simulink model "nonlin_3d"  (R2023a)
settings: Solver=ode1  StartTime=0  StopTime=400  FixedStep=0.002  RelTol=1e-3
values from neighbouring files (symbols this model uses):
  B1 = [-kQ, -kQ, kQ, kQ ... (first row only)    [simulate_hover.m]
  B2 = [0, 0, 0 ... (first row only)    [simulate_hover.m]
  beta3d = 0.9    [loadResultData.m]    (also in simulate_hover.m; temp.m)
  cycleGain = 0.2    [simulate_hover.m]    (also in temp.m = 1)
  epsilon3d = 1    [loadResultData.m]    (also in simulate_hover.m; temp.m)
  I_xx = 0.0522    [simulate_hover.m]
  I_yy = 0.0522    [simulate_hover.m]
  I_zz = 0.1104    [simulate_hover.m]
  K = lqi(sys, Q, R)    [simulate_hover.m]
  k3d = 1.65    [loadResultData.m]    (also in simulate_hover.m; temp.m)
  kfr_p = 0.4*u2line/x5line    (= 0.285774113641)    [simulate_hover.m]
  kfr_r = 0.4*u1line/x4line    (= 0.285774113641)    [simulate_hover.m]
  kfr_y = 0.4*u3line/x6line    (= 0.0880063173321)    [simulate_hover.m]
  sigma = 0    [simulate_hover.m]
  velMax = 100*60*pi/180    (= 104.71975512)    [simulate_hover.m]
  VMAX_AMP = 24    [setup_lab_hover.m]    (also in simulate_hover.m)
  wcf = 2 * pi * 20    (= 125.663706144)    [setup_lab_hover.m]    (also in simulate_hover.m)
  zetaf = 0.6    [setup_lab_hover.m]    (also in simulate_hover.m)
undefined symbols (not defined in the file or in its folder): DG
libraries: simulink_extras x1, dspsrcs4 x1
settings Model: Creator=kille  LastModifiedBy=Jacob

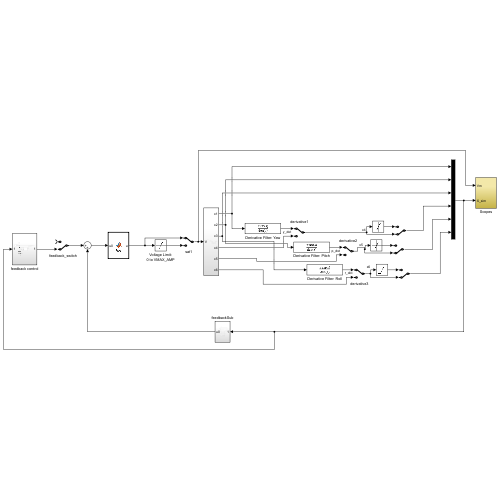
[thumbnail: Simulink's stored preview of the top-level diagram]
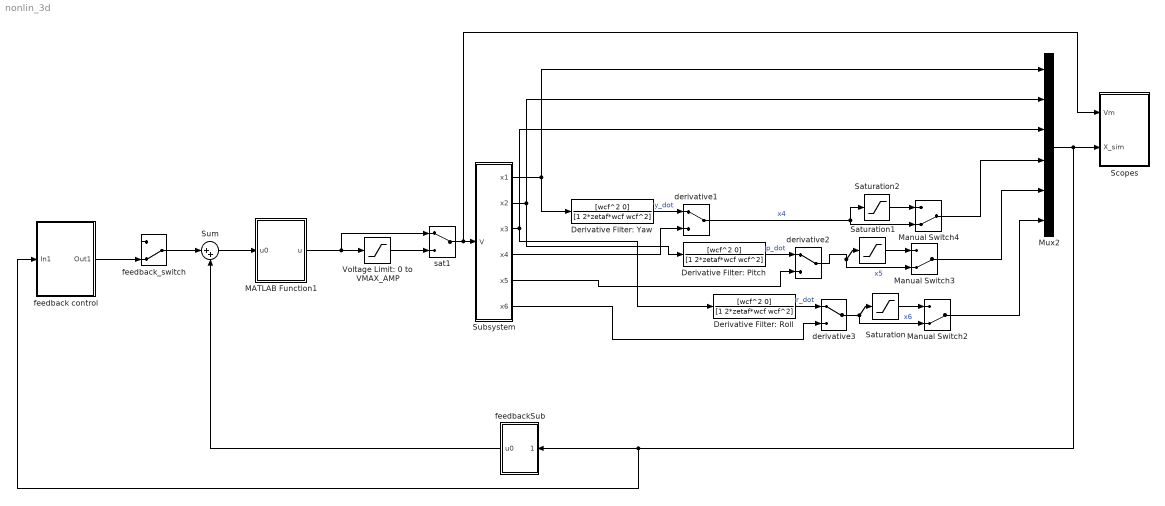
== system nonlin_3d ==
  Derivative Filter: Pitch : TransferFcn  Numerator=[wcf^2 0]  Denominator=[1 2*zetaf*wcf wcf^2]
  Derivative Filter: Roll : TransferFcn  Numerator=[wcf^2 0]  Denominator=[1 2*zetaf*wcf wcf^2]
  Derivative Filter: Yaw : TransferFcn  Numerator=[wcf^2 0]  Denominator=[1 2*zetaf*wcf wcf^2]
  MATLAB Function1 : MATLAB Function  TreatAsAtomicUnit=on
  Manual Switch2 : ManualSwitch  CurrentSetting=0
  Manual Switch3 : ManualSwitch  CurrentSetting=0
  Manual Switch4 : ManualSwitch  CurrentSetting=0
  Mux2 : Mux  Inputs=6
  Saturation : Saturate  UpperLimit=velMax  LowerLimit=-velMax
  Saturation1 : Saturate  UpperLimit=velMax  LowerLimit=-velMax
  Saturation2 : Saturate  UpperLimit=velMax  LowerLimit=-velMax
  Scopes : Subsystem
  Subsystem : Subsystem
  Sum : Sum  Inputs=|++
  Voltage Limit: 0 to VMAX_AMP : Saturate  UpperLimit=VMAX_AMP  LowerLimit=0
  derivative1 : ManualSwitch
  derivative2 : ManualSwitch
  derivative3 : ManualSwitch
  feedback control : Subsystem
  feedbackSub : Subsystem
  feedback_switch : ManualSwitch  CurrentSetting=0
  sat1 : ManualSwitch
  wires:
  Derivative Filter: Yaw/1 -> derivative1/1  "y_dot"
  Derivative Filter: Pitch/1 -> derivative2/1  "p_dot"
  Derivative Filter: Roll/1 -> derivative3/1  "r_dot"
  Subsystem/1(x1) -> Mux2/1, Derivative Filter: Yaw/1
  Subsystem/4(x4) -> derivative1/2
  Subsystem/2(x2) -> Derivative Filter: Pitch/1, Mux2/2
  Subsystem/5(x5) -> derivative2/2
  Subsystem/6(x6) -> derivative3/2
  Subsystem/3(x3) -> Mux2/3, Derivative Filter: Roll/1
  Manual Switch4/1 -> Mux2/4
  Manual Switch2/1 -> Mux2/6
  Manual Switch3/1 -> Mux2/5
  Saturation/1 -> Manual Switch2/1
  derivative3/1 -> Manual Switch2/2, Saturation/1  "x6"
  Saturation1/1 -> Manual Switch3/1
  derivative2/1 -> Manual Switch3/2, Saturation1/1  "x5"
  Saturation2/1 -> Manual Switch4/1
  derivative1/1 -> Saturation2/1, Manual Switch4/2  "x4"
  MATLAB Function1/1(u) -> sat1/1, Voltage Limit: 0 to VMAX_AMP/1
  sat1/1 -> Scopes/1(Vm), Subsystem/1(V)
  Voltage Limit: 0 to VMAX_AMP/1 -> sat1/2
  feedback control/1(Out1) -> feedback_switch/2
  Mux2/1 -> feedback control/1(In1), feedbackSub/1(Input), Scopes/2(X_sim)
  feedback_switch/1 -> Sum/1
  Sum/1 -> MATLAB Function1/1(u0)
  feedbackSub/1(u0) -> Sum/2

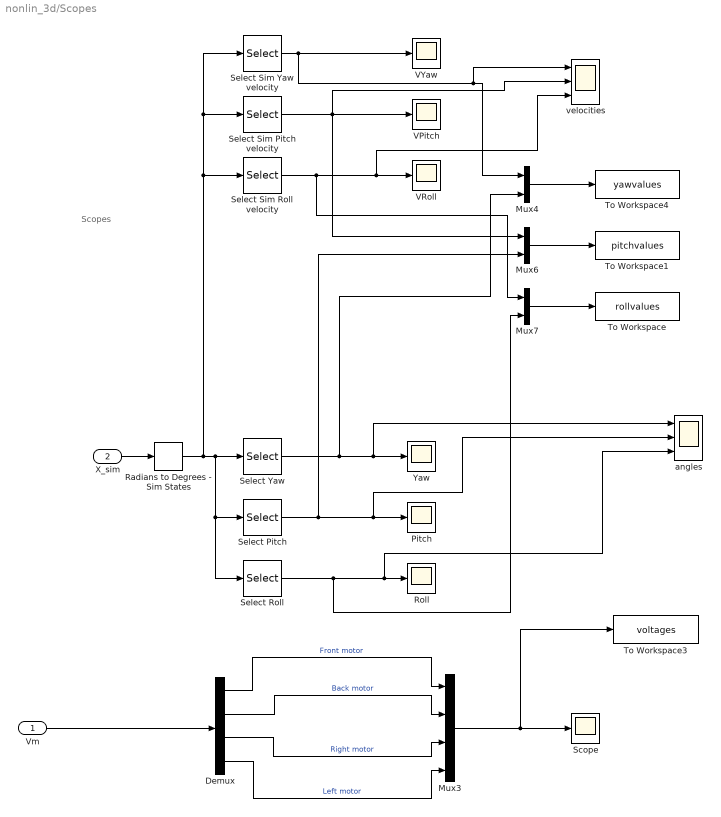
== system nonlin_3d/Scopes ==
  note: Scopes
  Vm : Inport
  X_sim : Inport  Port=2
  Demux : Demux
  Mux3 : Mux
  Mux4 : Mux  Inputs=2
  Mux6 : Mux  Inputs=2
  Mux7 : Mux  Inputs=2
  Pitch : Scope
  Radians to Degrees - Sim States : simulink_extras/Transformations/Radians to Degrees
  Roll : Scope
  Scope : Scope
  Select Pitch : Selector  InputPortWidth=6  IndexOptions=Index vector (dialog)  Indices=2  OutputSizes=1
  Select Roll : Selector  InputPortWidth=6  IndexOptions=Index vector (dialog)  Indices=3  OutputSizes=1
  Select Sim Pitch velocity : Selector  InputPortWidth=6  IndexOptions=Index vector (dialog)  Indices=5  OutputSizes=1
  Select Sim Roll velocity : Selector  InputPortWidth=6  IndexOptions=Index vector (dialog)  Indices=6  OutputSizes=1
  Select Sim Yaw velocity : Selector  InputPortWidth=6  IndexOptions=Index vector (dialog)  Indices=4  OutputSizes=1
  Select Yaw : Selector  InputPortWidth=6  IndexOptions=Index vector (dialog)  Indices=1  OutputSizes=1
  To Workspace : ToWorkspace  VariableName=rollvalues  SampleTime=-1
  To Workspace1 : ToWorkspace  VariableName=pitchvalues  SampleTime=-1
  To Workspace3 : ToWorkspace  VariableName=voltages  SampleTime=-1
  To Workspace4 : ToWorkspace  VariableName=yawvalues  SampleTime=-1
  VPitch : Scope
  VRoll : Scope
  VYaw : Scope
  Yaw : Scope
  angles : Scope  NumInputPorts=3
  velocities : Scope  NumInputPorts=3
  wires:
  Select Roll/1 -> angles/3, Roll/1, Mux7/2
  Radians to Degrees - Sim States/1 -> Select Sim Roll velocity/1, Select Sim Pitch velocity/1, Select Sim Yaw velocity/1, Select Roll/1, Select Pitch/1, Select Yaw/1
  Select Pitch/1 -> angles/2, Pitch/1, Mux6/2
  X_sim/1 -> Radians to Degrees - Sim States/1
  Demux/1 -> Mux3/1  "Front motor"
  Demux/2 -> Mux3/2  "Back motor"
  Demux/3 -> Mux3/3  "Right motor"
  Demux/4 -> Mux3/4  "Left motor"
  Vm/1 -> Demux/1
  Select Sim Yaw velocity/1 -> VYaw/1, velocities/1, Mux4/1
  Select Sim Roll velocity/1 -> velocities/3, VRoll/1, Mux7/1
  Select Sim Pitch velocity/1 -> Mux6/1, velocities/2, VPitch/1
  Mux4/1 -> To Workspace4/1
  Mux6/1 -> To Workspace1/1
  Mux7/1 -> To Workspace/1
  Mux3/1 -> To Workspace3/1, Scope/1
  Select Yaw/1 -> angles/1, Yaw/1, Mux4/2

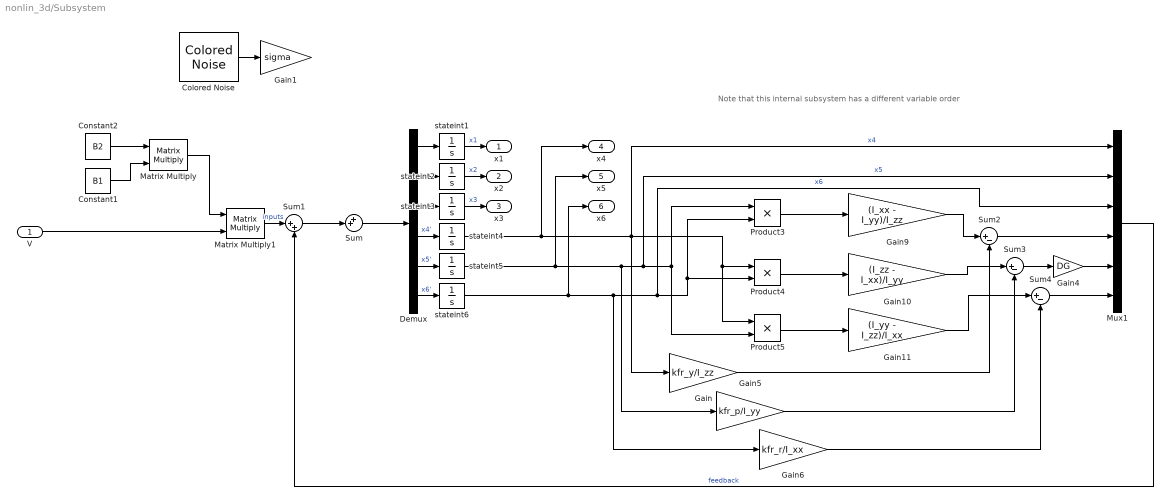
== system nonlin_3d/Subsystem ==
  note: Note that this internal subsystem has a different variable order
  V : Inport
  Colored Noise : dspsrcs4/Colored Noise  Color=white  InverseFrequencyPower=1  BoundedOutput=off  NumChannels=6  OutputDataType=double  SamplesPerFrame=1  SampleTime=1  RandomStream=mt19937ar with seed  Seed=67  SimulateUsing=Interpreted execution
  Constant1 : Constant  Value=B1
  Constant2 : Constant  Value=B2
  Demux : Demux  Outputs=6
  Gain : Gain  Gain=kfr_y/I_zz
  Gain1 : Gain  Gain=sigma
  Gain10 : Gain  Gain=(I_zz - I_xx)/I_yy
  Gain11 : Gain  Gain=(I_yy - I_zz)/I_xx
  Gain4 : Gain  Gain=DG
  Gain5 : Gain  Gain=kfr_p/I_yy
  Gain6 : Gain  Gain=kfr_r/I_xx
  Gain9 : Gain  Gain=(I_xx - I_yy)/I_zz
  Matrix Multiply : Product  Multiplication=Matrix(*)
  Matrix Multiply1 : Product  Multiplication=Matrix(*)
  Mux1 : Mux  Inputs=6
  Product3 : Product
  Product4 : Product
  Product5 : Product
  Sum : Sum  Inputs=++|
  Sum1 : Sum  Inputs=|++
  Sum2 : Sum  Inputs=|+-
  Sum3 : Sum  Inputs=|+-
  Sum4 : Sum  Inputs=|+-
  stateint{1,4..6} (4 alike) : Integrator
  stateint2 : Integrator  InitialCondition=0.00010472
  stateint3 : Integrator  InitialCondition=0.00010472
  x1 : Outport
  x2 : Outport  Port=2
  x3 : Outport  Port=3
  x4 : Outport  Port=4
  x5 : Outport  Port=5
  x6 : Outport  Port=6
  wires:
  Mux1/1 -> Sum1/2  "feedback"
  stateint5/1 -> x5/1, Gain5/1, Mux1/2, Product5/2, Product3/1  "x5"
  Matrix Multiply1/1 -> Sum1/1  "inputs"
  stateint4/1 -> x4/1, Gain/1, Mux1/1, Product5/1, Product4/1  "x4"
  Matrix Multiply/1 -> Matrix Multiply1/1
  V/1 -> Matrix Multiply1/2
  Sum2/1 -> Mux1/4
  Gain6/1 -> Sum4/2
  Demux/1 -> stateint1/1
  stateint6/1 -> x6/1, Gain6/1, Mux1/3, Product4/2, Product3/2  "x6"
  Demux/6 -> stateint6/1  "x6'"
  Product5/1 -> Gain11/1
  Demux/5 -> stateint5/1  "x5'"
  Demux/2 -> stateint2/1
  Gain11/1 -> Sum4/1
  Constant1/1 -> Matrix Multiply/2
  Demux/3 -> stateint3/1
  Gain9/1 -> Sum2/1
  Gain10/1 -> Sum3/1
  Constant2/1 -> Matrix Multiply/1
  Demux/4 -> stateint4/1  "x4'"
  Product4/1 -> Gain10/1
  stateint1/1 -> x1/1  "x1"
  stateint2/1 -> x2/1  "x2"
  stateint3/1 -> x3/1  "x3"
  Colored Noise/1 -> Gain1/1
  Sum1/1 -> Sum/2
  Sum/1 -> Demux/1
  Product3/1 -> Gain9/1
  Gain/1 -> Sum2/2
  Gain5/1 -> Sum3/2
  Sum3/1 -> Gain4/1
  Sum4/1 -> Mux1/6
  Gain4/1 -> Mux1/5

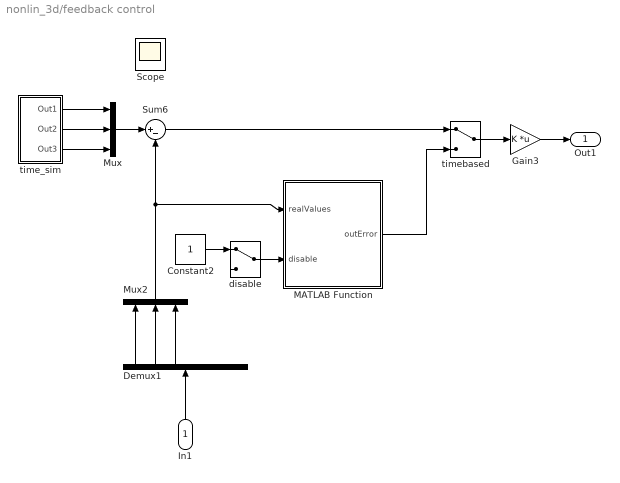
== system nonlin_3d/feedback control ==
  In1 : Inport
  Constant2 : Constant
  Demux1 : Demux  Outputs=6
  Gain3 : Gain  Gain=K  Multiplication=Matrix(K*u)
  MATLAB Function : MATLAB Function  TreatAsAtomicUnit=on
  Mux : Mux  Inputs=3
  Mux2 : Mux  Inputs=3
  Scope : Scope
  Sum6 : Sum  Inputs=|+-
  disable : ManualSwitch
  time_sim : Subsystem
  timebased : ManualSwitch
  Out1 : Outport
  wires:
  Demux1/2 -> Mux2/2
  Demux1/1 -> Mux2/1
  Demux1/3 -> Mux2/3
  In1/1 -> Demux1/1
  MATLAB Function/1(outError) -> timebased/2
  Sum6/1 -> timebased/1
  timebased/1 -> Gain3/1
  Gain3/1 -> Out1/1
  Mux2/1 -> MATLAB Function/1(realValues), Sum6/2
  disable/1 -> MATLAB Function/2(disable)
  Constant2/1 -> disable/1
  Mux/1 -> Sum6/1
  time_sim/1(Out1) -> Mux/1
  time_sim/2(Out2) -> Mux/2
  time_sim/3(Out3) -> Mux/3

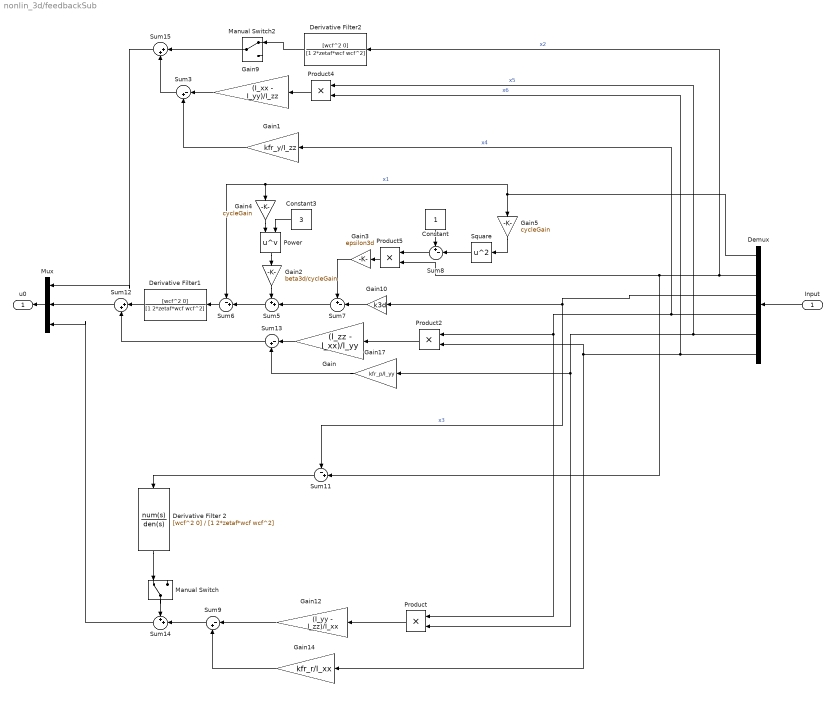
== system nonlin_3d/feedbackSub ==
  Input : Inport
  Constant : Constant
  Constant3 : Constant  Value=3
  Demux : Demux  Outputs=6
  Derivative Filter 2 : TransferFcn  Numerator=[wcf^2 0]  Denominator=[1 2*zetaf*wcf wcf^2]
  Derivative Filter1 : TransferFcn  Numerator=[wcf^2 0]  Denominator=[1 2*zetaf*wcf wcf^2]
  Derivative Filter2 : TransferFcn  Numerator=[wcf^2 0]  Denominator=[1 2*zetaf*wcf wcf^2]
  Gain : Gain  Gain=(I_zz - I_xx)/I_yy
  Gain1 : Gain  Gain=kfr_y/I_zz
  Gain10 : Gain  Gain=k3d
  Gain12 : Gain  Gain=(I_yy - I_zz)/I_xx
  Gain14 : Gain  Gain=kfr_r/I_xx
  Gain17 : Gain  Gain=kfr_p/I_yy
  Gain2 : Gain  Gain=beta3d/cycleGain
  Gain3 : Gain  Gain=epsilon3d
  Gain4 : Gain  Gain=cycleGain
  Gain5 : Gain  Gain=cycleGain
  Gain9 : Gain  Gain=(I_xx - I_yy)/I_zz
  Manual Switch : ManualSwitch
  Manual Switch2 : ManualSwitch
  Mux : Mux  Inputs=3
  Power : Math  Operator=pow
  Product{,2,4..5} (4 alike) : Product
  Square : Math  Operator=square
  Sum11 : Sum  Inputs=-+|
  Sum12 : Sum  Inputs=|++
  Sum13 : Sum  Inputs=|-+
  Sum14 : Sum  Inputs=++|
  Sum15 : Sum  Inputs=|++
  Sum3 : Sum  Inputs=|-+
  Sum5 : Sum  Inputs=++|
  Sum6 : Sum  Inputs=-+|
  Sum7 : Sum  Inputs=+-|
  Sum8 : Sum  Inputs=+-|
  Sum9 : Sum  Inputs=|-+
  u0 : Outport
  wires:
  Gain17/1 -> Sum13/2
  Sum13/1 -> Sum12/2
  Demux/4 -> Product/1, Product2/1, Gain1/1  "x4"
  Product2/1 -> Gain/1
  Demux/5 -> Product4/1, Product/2, Gain17/1  "x5"
  Product/1 -> Gain12/1
  Demux/6 -> Gain14/1, Product2/2, Product4/2  "x6"
  Manual Switch/1 -> Sum14/1
  Sum9/1 -> Sum14/2
  Gain12/1 -> Sum9/1
  Gain/1 -> Sum13/1
  Gain14/1 -> Sum9/2
  Sum12/1 -> Mux/2
  Derivative Filter 2/1 -> Manual Switch/1
  Sum14/1 -> Mux/3
  Input/1 -> Demux/1
  Demux/3 -> Gain10/1, Sum11/1  "x3"
  Product4/1 -> Gain9/1
  Gain9/1 -> Sum3/1
  Gain1/1 -> Sum3/2
  Gain3/1 -> Sum7/1
  Gain2/1 -> Sum5/1
  Constant/1 -> Sum8/1
  Constant3/1 -> Power/2
  Square/1 -> Sum8/2
  Sum8/1 -> Product5/1
  Gain10/1 -> Sum7/2
  Sum7/1 -> Sum5/2
  Sum5/1 -> Sum6/2
  Product5/1 -> Gain3/1
  Power/1 -> Gain2/1
  Manual Switch2/1 -> Sum15/1
  Demux/2 -> Derivative Filter2/1, Product5/2, Sum11/2  "x2"
  Derivative Filter2/1 -> Manual Switch2/1
  Sum3/1 -> Sum15/2
  Demux/1 -> Gain4/1, Sum6/1, Gain5/1  "x1"
  Derivative Filter1/1 -> Sum12/1
  Sum6/1 -> Derivative Filter1/1
  Sum11/1 -> Derivative Filter 2/1
  Sum15/1 -> Mux/1
  Mux/1 -> u0/1
  Gain4/1 -> Power/1
  Gain5/1 -> Square/1

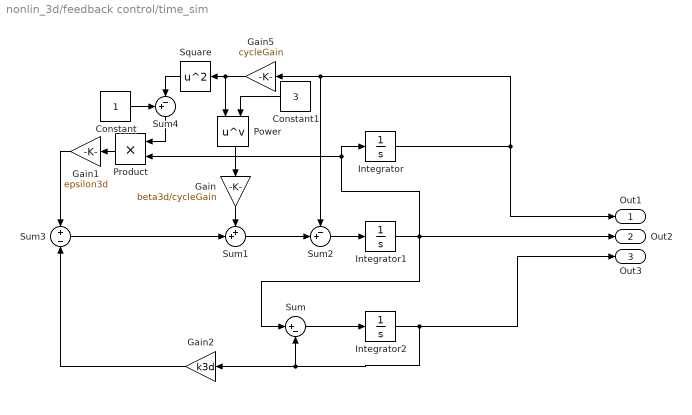
== system nonlin_3d/feedback control/time_sim ==
  Constant : Constant
  Constant1 : Constant  Value=3
  Gain : Gain  Gain=beta3d/cycleGain
  Gain1 : Gain  Gain=epsilon3d
  Gain2 : Gain  Gain=k3d
  Gain5 : Gain  Gain=cycleGain
  Integrator : Integrator  InitialCondition=0.0001
  Integrator1 : Integrator  InitialCondition=0.0001
  Integrator2 : Integrator  InitialCondition=0.0001
  Power : Math  Operator=pow
  Product : Product
  Square : Math  Operator=square
  Sum : Sum  Inputs=|+-
  Sum1 : Sum  Inputs=++|
  Sum2 : Sum  Inputs=-+|
  Sum3 : Sum  Inputs=+|-
  Sum4 : Sum  Inputs=+-|
  Out1 : Outport
  Out2 : Outport  Port=2
  Out3 : Outport  Port=3
  wires:
  Gain5/1 -> Square/1, Power/1
  Integrator1/1 -> Out2/1, Sum/1, Product/2, Integrator/1
  Constant/1 -> Sum4/1
  Integrator2/1 -> Out3/1, Sum/2, Gain2/1
  Gain/1 -> Sum1/1
  Square/1 -> Sum4/2
  Integrator/1 -> Out1/1, Sum2/1, Gain5/1
  Sum2/1 -> Integrator1/1
  Sum1/1 -> Sum2/2
  Power/1 -> Gain/1
  Sum4/1 -> Product/1
  Sum3/1 -> Sum1/2
  Sum/1 -> Integrator2/1
  Gain1/1 -> Sum3/1
  Constant1/1 -> Power/2
  Product/1 -> Gain1/1
  Gain2/1 -> Sum3/2

== matlab function nonlin_3d/feedback control/MATLAB Function ==
  data: realValues input; outError output; disable input
function outError = approxLimitSimu(realValues, disable)
    outError = transpose([0, 0, 0]);
    %temp = load('paperCycle.mat');
    %cycleValues = temp.paperCycle;
    %for n = 1:2
    %    cycleN = cycleValues(:, n);
    %    realValueN = realValues(n);
    %    [closestValueError,idx]=min(abs(cycleN-realValueN));
    %    outError(n) = closestValueError;
    %end
    %disp(length(cycleValues))
    coder.extrinsic('approxLimit');
    if disable ~= 1
        outError = transpose(approxLimit(realValues));
    end

== matlab function nonlin_3d/MATLAB Function1 ==
  data: u output; u0 input
function u = fcn(u0)
    % %x1, x2, x3, x4, x5, x6 = x;
    % uG1 = 0;
    % uG2 = 0;
    u1 = 0;
    u2 = 0;
    u3 = 0;
    u4 = 0;

    coder.extrinsic('solveSyms3d_2');
    % coder.extrinsic('solveSyms4');
    % if x5 ~= 0 & x6 ~= 0
    %     [u1, u2, u3, u4] = solveSyms4(x5, x6, u0(1), u0(2), u0(3));
    % else
    %     u1 = 0.01;
    %     u2 = 0.01;
    %     u3 = 0.01;
    %     u4 = 0.01;
    % 
    % end
    [u1, u2, u3, u4] = solveSyms3d_2(u0(1), u0(2), u0(3));
    u = transpose([u1 + 12, u2 + 12, u3 + 12, u4 + 12]);
    %u = transpose([u1, 12, u2, 12]);


end
